simulink model "Single_Boiler_Model"  (R2025b)
settings: Solver=ode15s  StartTime=0.0  StopTime=180  FixedStep=1000  RelTol=1e-2
values from neighbouring files (symbols this model uses):
  Adc = 0.7    [INIT_BOILER.m]
  b = 0.030e2    (= 3)    [INIT_BOILER.m]
  k1 = circ_numerator / (qdc0_target^2)    [INIT_BOILER.m]
  m_metal = 0.3*(1e6)    (= 300000)    [INIT_BOILER.m]
  m_riser = 2.0e5    (= 200000)    [INIT_BOILER.m]
  tau_s = 1e-2    (= 0.01)    [INIT_BOILER.m]
  u0 = [Q0_MW; qf0; qs0; hf0]    [INIT_BOILER.m]
  Vr = 37    [INIT_BOILER.m]
  x0 = [Vwt0; p0_MPa; a30; Vsd0]    [INIT_BOILER.m]
settings Model: SimulationMode=accelerator  PacingRate=100  Creator=Zwivh  LastModifiedBy=Zwivh

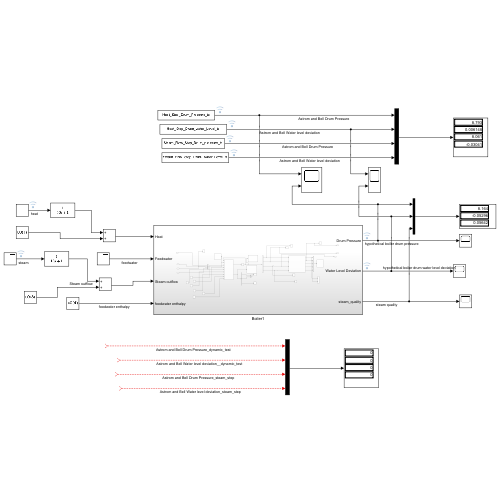
[thumbnail: Simulink's stored preview of the top-level diagram]
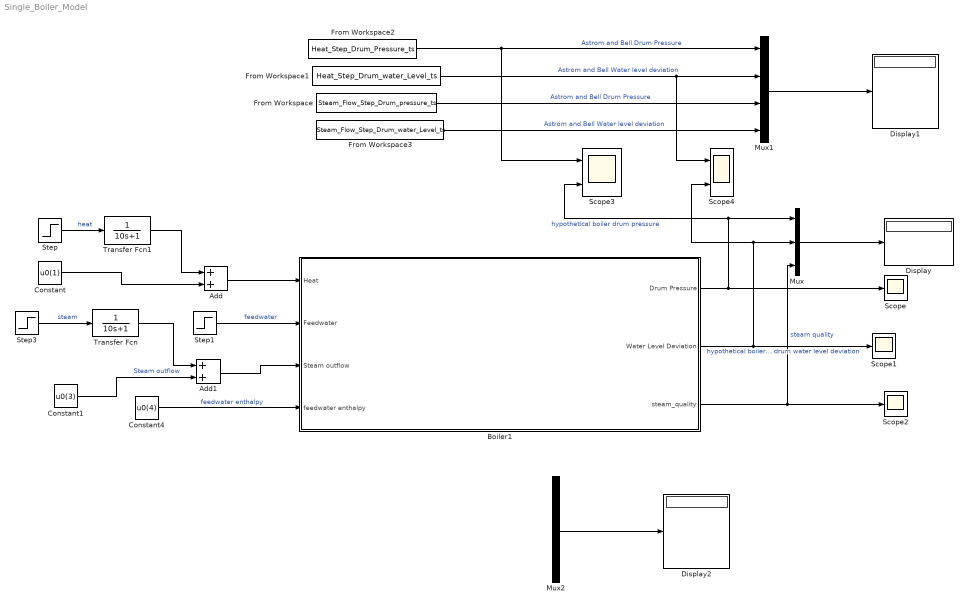
== system Single_Boiler_Model ==
  Add : Sum
  Add1 : Sum
  Boiler1 : Subsystem
  Constant : Constant  Value=u0(1)
  Constant1 : Constant  Value=u0(3)
  Constant4 : Constant  Value=u0(4)
  Display : Display
  Display1 : Display
  Display2 : Display
  From Workspace : FromWorkspace  VariableName=Steam_Flow_Step_Drum_pressure_ts
  From Workspace1 : FromWorkspace  VariableName=Heat_Step_Drum_water_Level_ts
  From Workspace2 : FromWorkspace  VariableName=Heat_Step_Drum_Pressure_ts
  From Workspace3 : FromWorkspace  VariableName=Steam_Flow_Step_Drum_water_Level_ts
  Mux : Mux  Inputs=3
  Mux1 : Mux
  Mux2 : Mux
  Scope : Scope
      settings: DataLoggingVariableName=ScopeData7
  Scope1 : Scope
      settings: ActiveDisplayYMinimum=-1  ActiveDisplayYMaximum=1  DataLoggingVariableName=ScopeData10
  Scope2 : Scope
      settings: DataLoggingVariableName=ScopeData11
  Scope3 : Scope  NumInputPorts=2
      settings: ActiveDisplayYMinimum=8.4630372129045046  ActiveDisplayYMaximum=8.8300659694282047  DataLoggingVariableName=ScopeData12
  Scope4 : Scope  NumInputPorts=2
      settings: DataLoggingVariableName=ScopeData13
  Step : Step  Time=500  After=u0(1)*0.1  SampleTime=0
  Step1 : Step  Time=50  Before=u0(2)  After=u0(2)+00  SampleTime=0
  Step3 : Step  Time=50  After=u0(3)*0.1-u0(3)*0.1  SampleTime=0
  Transfer Fcn : TransferFcn  Denominator=[10 1]
  Transfer Fcn1 : TransferFcn  Denominator=[10 1]
  wires:
  Mux/1 -> Display/1
  Boiler1/1(Drum Pressure) -> Scope3/2, Mux/1, Scope/1  "hypothetical boiler drum pressure"
  Boiler1/3(steam_quality) -> Mux/3, Scope2/1  "steam quality"
  Constant4/1 -> Boiler1/4(feedwater enthalpy)  "feedwater enthalpy"
  Step/1 -> Transfer Fcn1/1  "heat"
  Step1/1 -> Boiler1/2(Feedwater)  "feedwater"
  Boiler1/2(Water Level Deviation) -> Scope4/2, Mux/2, Scope1/1  "hypothetical boiler drum water level deviation"
  Constant1/1 -> Add1/2  "Steam outflow"
  Add/1 -> Boiler1/1(Heat)
  Constant/1 -> Add/2
  Step3/1 -> Transfer Fcn/1  "steam"
  Add1/1 -> Boiler1/3(Steam outflow)
  From Workspace2/1 -> Scope3/1, Mux1/1  "Astrom and Bell Drum Pressure"
  From Workspace1/1 -> Scope4/1, Mux1/2  "Astrom and Bell Water level deviation"
  From Workspace/1 -> Mux1/3  "Astrom and Bell Drum Pressure"
  Mux1/1 -> Display1/1
  From Workspace3/1 -> Mux1/4  "Astrom and Bell Water level deviation"
  Mux2/1 -> Display2/1
  ? -> Mux2/4  "Astrom and Bell Water level deviation_steam_step"
  ? -> Mux2/2  "Astrom and Bell Water level deviation__dynamic_test"
  ? -> Mux2/3  "Astrom and Bell Drum Pressure_steam_step"
  ? -> Mux2/1  "Astrom and Bell Drum Pressure_dynamic_test"
  Transfer Fcn/1 -> Add1/1
  Transfer Fcn1/1 -> Add/1

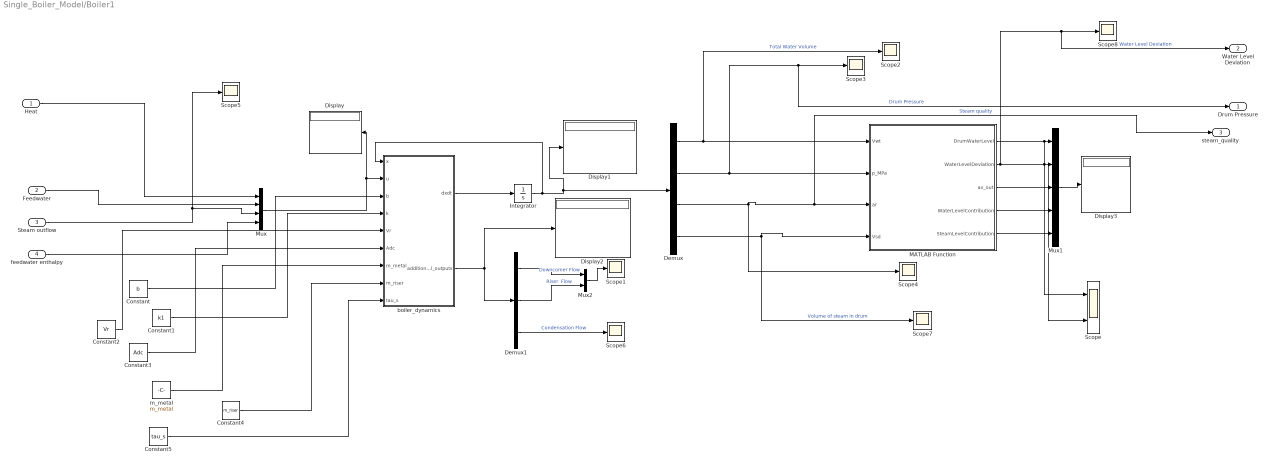
== system Single_Boiler_Model/Boiler1 ==
  Heat : Inport
  Feedwater : Inport  Port=2
  Steam outflow : Inport  Port=3
  feedwater enthalpy : Inport  Port=4
  Constant : Constant  Value=b
  Constant1 : Constant  Value=k1
  Constant2 : Constant  Value=Vr
  Constant3 : Constant  Value=Adc
  Constant4 : Constant  Value=m_riser
  Constant5 : Constant  Value=tau_s
  Demux : Demux
  Demux1 : Demux  Outputs=3
  Display{,1..3} (4 alike) : Display
  Integrator : Integrator  InitialCondition=x0
  MATLAB Function : MATLAB Function  TreatAsAtomicUnit=on
  Mux : Mux
  Mux1 : Mux  Inputs=5
  Mux2 : Mux  Inputs=2
  Scope : Scope  NumInputPorts=2
      settings: ActiveDisplayYMinimum=-0.11553187271684388  ActiveDisplayYMaximum=0.97989716685186512  DataLoggingVariableName=ScopeData9
  Scope{1..8} (8 alike) : Scope
      Scope1 settings: ActiveDisplayYMinimum=1149.8937170235527  ActiveDisplayYMaximum=1360.0825647224879  DataLoggingVariableName=ScopeData6
      Scope3 settings: ActiveDisplayYMinimum=5.1731172032500083  ActiveDisplayYMaximum=8.869653644083332
      Scope4 settings: DataLoggingVariableName=ScopeData2
      Scope5 settings: ActiveDisplayYMinimum=81.783639946245515  ActiveDisplayYMaximum=87.68969538020076  DataLoggingVariableName=ScopeData3
      Scope6 settings: DataLoggingVariableName=ScopeData4
      Scope7 settings: DataLoggingVariableName=ScopeData5
      Scope8 settings: ActiveDisplayYMinimum=-0.31931831052985321  ActiveDisplayYMaximum=0.12332586369569878  DataLoggingVariableName=ScopeData8
  boiler_dynamics : MATLAB Function  TreatAsAtomicUnit=on
  "m_metal " : Constant  Value=m_metal
  Drum Pressure : Outport
  Water Level Deviation : Outport  Port=2
  steam_quality : Outport  Port=3
  wires:
  MATLAB Function/3(av_out) -> Mux1/3
  Steam outflow/1 -> Scope5/1, Mux/3
  Integrator/1 -> Display1/1, Demux/1, boiler_dynamics/1(x)
  Constant4/1 -> boiler_dynamics/8(m_riser)
  Demux/1 -> Scope2/1, MATLAB Function/1(Vwt)  "Total Water Volume"
  MATLAB Function/2(WaterLevelDeviation) -> Water Level Deviation/1, Scope8/1, Scope/2, Mux1/2  "Water Level Deviation"
  Demux/2 -> Drum Pressure/1, Scope3/1, MATLAB Function/2(p_MPa)  "Drum Pressure"
  Demux1/2 -> Mux2/2  "Riser  Flow"
  boiler_dynamics/2(additional_outputs) -> Display2/1, Demux1/1
  Constant2/1 -> boiler_dynamics/5(Vr)
  Demux/3 -> Scope4/1, steam_quality/1, MATLAB Function/3(ar)  "Steam quality"
  Constant3/1 -> boiler_dynamics/6(Adc)
  Mux2/1 -> Scope1/1
  Demux1/1 -> Mux2/1  "Downcomer Flow"
  Constant1/1 -> boiler_dynamics/4(k)
  Mux/1 -> Display/1, boiler_dynamics/2(u)
  MATLAB Function/5(SteamLevelContribution) -> Mux1/5
  MATLAB Function/1(DrumWaterLevel) -> Scope/1, Mux1/1
  Constant/1 -> boiler_dynamics/3(b)
  "m_metal "/1 -> boiler_dynamics/7(m_metal)
  Demux/4 -> Scope7/1, MATLAB Function/4(Vsd)  "Volume of steam in drum"
  Constant5/1 -> boiler_dynamics/9(tau_s)
  Heat/1 -> Mux/1
  boiler_dynamics/1(dxdt) -> Integrator/1
  Demux1/3 -> Scope6/1  "Condensation Flow"
  MATLAB Function/4(WaterLevelContribution) -> Mux1/4
  Mux1/1 -> Display3/1
  Feedwater/1 -> Mux/2
  feedwater enthalpy/1 -> Mux/4

== matlab function Single_Boiler_Model/Boiler1/MATLAB Function ==
  data: Vwt input; DrumWaterLevel output; p_MPa input; ar input; Vsd input; WaterLevelDeviation output; av_out output; WaterLevelContribution output; SteamLevelContribution output
function [DrumWaterLevel, WaterLevelDeviation, av_out, WaterLevelContribution, SteamLevelContribution] = drum_level(Vwt, p_MPa, ar, Vsd)


[DrumWaterLevel, WaterLevelDeviation, av_out, WaterLevelContribution, SteamLevelContribution] = calculate_level(Vwt, p_MPa, ar, Vsd)

== matlab function Single_Boiler_Model/Boiler1/boiler_dynamics ==
  data: x input size=[4 1]; u input size=[4 1]; b input size=[1 1]; k input size=[1 1]; Vr input size=[1 1]; Adc input size=[1 1]; m_metal input size=[1 1]; m_riser input size=[1 1]; dxdt output size=[4 1]; tau_s input size=[1 1]; additional_outputs output size=[6 1]
function [dxdt, additional_outputs] = boiler(x, u, b, k, Vr, Adc, m_metal, m_riser, tau_s)
%#codegen
% Wrapper that calls the external boiler dynamics function.
[dxdt, additional_outputs] = boiler_dynamics_block( ...
    x, u, b, k, Vr, Adc, m_metal, m_riser, tau_s );
